simulink model "sim_tutorial2"  (Simulink 3.00)
settings: Solver=ode23tb  StartTime=0.0  StopTime=100  RelTol=1e-3  AbsTol=1e-4
values from neighbouring files (symbols this model uses):
  Rot = rotfe(Rot)    [tst_frf1.m]    (also in tst_reduce1.m; tst_sim1.m)
undefined symbols (not defined in the file or in its folder): a, b, bu, c, d, du
libraries: simulink3 x3

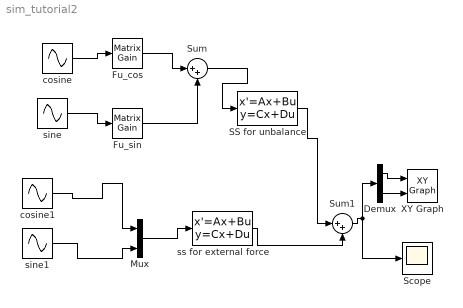
== system sim_tutorial2 ==
  Demux : Demux  Outputs=2
  Fu_cos : simulink3/Math/Matrix Gain  K=Rot.Fu_cos
  Fu_sin : simulink3/Math/Matrix Gain  K=Rot.Fu_sin
  Mux : Mux  Inputs=2
  SS for unbalance : StateSpace  A=a  B=bu  C=c  D=du  X0=0
  Scope : Scope
      settings: TimeRange=auto  YMin=-0.01  YMax=0.0125  SaveToWorkspace=off  SaveName=ScopeData
  Sum : Sum  Inputs=|++  SaturateOnIntegerOverflow=on
  Sum1 : Sum  Inputs=|++  SaturateOnIntegerOverflow=on
  XY Graph : simulink3/Sinks/XY Graph  xmin=-1e-2  xmax=1e-2  ymin=-1e-2  ymax=1e-2  st=-1
  cosine : Sin  Amplitude=1  Frequency=Rot.W  Phase=pi/2  SampleTime=0
  cosine1 : Sin  Amplitude=1  Frequency=1.21  Phase=pi/2  SampleTime=0
  sine : Sin  Amplitude=1  Frequency=Rot.W  Phase=0  SampleTime=0
  sine1 : Sin  Amplitude=1  Frequency=1  Phase=0  SampleTime=0
  ss for external force : StateSpace  A=a  B=b  C=c  D=d  X0=0
  wires:
  cosine/1 -> Fu_cos/1
  sine/1 -> Fu_sin/1
  Sum/1 -> SS for unbalance/1
  Fu_cos/1 -> Sum/1
  Fu_sin/1 -> Sum/2
  Mux/1 -> ss for external force/1
  ss for external force/1 -> Sum1/2
  Sum1/1 -> Scope/1, Demux/1
  Demux/2 -> XY Graph/2
  Demux/1 -> XY Graph/1
  SS for unbalance/1 -> Sum1/1
  sine1/1 -> Mux/2
  cosine1/1 -> Mux/1
